simulink model "EV_PV_Charging"  (R2025a)
settings: Solver=ode3  StartTime=0.0  StopTime=1  RelTol=1e-3
PreLoadFcn:
  | %% Parameter file: OBC_4_data.m
  | 
  | %% Model Parameters
  | Ts_Power= 50e-9;        % SPS Model sample time (s)
  | Co=150e-6;              % Output filter (F)
  | Ron_FET=50e-3;          % FET resistance (ohms)
  | Ron_Diode=50e-3;        % FET resistance (ohms)
  | Vf=0.6;                 % Diode forward voltage (V)
  | %
  | %% PFC Data
  | Vnom_ac= 240;           % Nominal Ac voltage (V)
  | Fnom= 60;               % System frequency (Hz)
  | L_PFC= 600e-6;          % PFC Inductance (H)
  | RL_PFC= 20e-3;          % Inductance resistance (Ohm)
  | C_PFC= 2600e-6;         % Capacitance (F)
  | 
  | %% PFC Control System Parameters
  | Ts_Control= 10e-6;      % Control system time (s)
  | Fsw= 100e3;             % PWM Switching frequency (Hz)
  | DT_PFC=400e-9;
  | %
  | % Current Regulator (PR):
  | Kp_I= 0.06;             % Proportional gain
  | Kr_I= 2.5;              % Resonant gain
  | Zeta_I=0.2;             % Damping coefficient
  | Fr_I=Fnom*2;            % Resonant frequency (Hz)
  | %
  | % Voltage Regulator (PI):
  | Kp_V= 0.25;             % Proportional gain
  | Ki_V= 80;               % Integral gain
  | Limit_V= 100;           % Output limit
  | %
  | %% LLC Data
  | Vdc_in=400;             % DC input voltage (V)
  | Vo_nom=400;             % DC nominal output voltage (V)
  | Po_nom=7.2e3;           % Nominal output power (W)
  | Lr=25e-6;               % Transformer leakage inductance (Resonant inductance in Henry)
  | Lm=150e-6;              % Magnetization inductance (H)
  | Cr=75e-9;               % Resonant capacitor (F)
  | Np=10; Ns=12; N=Np/Ns;  % Transformer ratio
  | %
  | %% LLC Control System Parameters
  | DT_LLC=400e-9;
  | Ts_Control=10e-6;
  | % Voltage Regulator (PI):
  | Kp_LLC= 100/4;          % Proportional gain
  | Ki_LLC= 150e3;          % Integral gain
  | fs_LCC_min= 120e3;      % Minimum switching frequency (Hz)
  | fs_LCC_max= 300e3;      % Maximum switching frequency (Hz)
  | Vref_LCC_min= 275;      % Minimum voltage setpoint (V)
  | Vref_LCC_max= 450;      % Maximum voltage setpoint (V)
  | %
  | %%
  | % Resonant tank data
  | Ro=Vo_nom^2/Po_nom      % LLC output load (Ohm)
  | Rac=(8/pi^2)*N^2*Ro     % Equivalent pprimary AC resistance (Ohm)
  | Q=sqrt(Lr/Cr)/Rac       % Quality factor
  | fr=1/(2*pi*sqrt(Lr*Cr)) % Resonant frequency (Hz)
  | m=(Lr+Lm)/Lr            % Ratio of total primary reactance to resonant inductance (Lr)
  | %%
InitFcn:
  | %% Parameter file: OBC_4_data.m
  | 
  | %% Model Parameters
  | Ts_Power= 50e-9;        % SPS Model sample time (s)
  | Co=150e-6;              % Output filter (F)
  | Ron_FET=50e-3;          % FET resistance (ohms)
  | Ron_Diode=50e-3;        % FET resistance (ohms)
  | Vf=0.6;                 % Diode forward voltage (V)
  | %
  | %% PFC Data
  | Vnom_ac= 240;           % Nominal Ac voltage (V)
  | Fnom= 60;               % System frequency (Hz)
  | L_PFC= 600e-6;          % PFC Inductance (H)
  | RL_PFC= 20e-3;          % Inductance resistance (Ohm)
  | C_PFC= 2600e-6;         % Capacitance (F)
  | 
  | %% PFC Control System Parameters
  | Ts_Control= 10e-6;      % Control system time (s)
  | Fsw= 100e3;             % PWM Switching frequency (Hz)
  | DT_PFC=400e-9;
  | %
  | % Current Regulator (PR):
  | Kp_I= 0.06;             % Proportional gain
  | Kr_I= 2.5;              % Resonant gain
  | Zeta_I=0.2;             % Damping coefficient
  | Fr_I=Fnom*2;            % Resonant frequency (Hz)
  | %
  | % Voltage Regulator (PI):
  | Kp_V= 0.25;             % Proportional gain
  | Ki_V= 80;               % Integral gain
  | Limit_V= 100;           % Output limit
  | %
  | %% LLC Data
  | Vdc_in=400;             % DC input voltage (V)
  | Vo_nom=400;             % DC nominal output voltage (V)
  | Po_nom=7.2e3;           % Nominal output power (W)
  | Lr=25e-6;               % Transformer leakage inductance (Resonant inductance in Henry)
  | Lm=150e-6;              % Magnetization inductance (H)
  | Cr=75e-9;               % Resonant capacitor (F)
  | Np=10; Ns=12; N=Np/Ns;  % Transformer ratio
  | %
  | %% LLC Control System Parameters
  | DT_LLC=400e-9;
  | Ts_Control=10e-6;
  | % Voltage Regulator (PI):
  | Kp_LLC= 100/4;          % Proportional gain
  | Ki_LLC= 150e3;          % Integral gain
  | fs_LCC_min= 120e3;      % Minimum switching frequency (Hz)
  | fs_LCC_max= 300e3;      % Maximum switching frequency (Hz)
  | Vref_LCC_min= 275;      % Minimum voltage setpoint (V)
  | Vref_LCC_max= 450;      % Maximum voltage setpoint (V)
  | %
  | %%
  | % Resonant tank data
  | Ro=Vo_nom^2/Po_nom      % LLC output load (Ohm)
  | Rac=(8/pi^2)*N^2*Ro     % Equivalent pprimary AC resistance (Ohm)
  | Q=sqrt(Lr/Cr)/Rac       % Quality factor
  | fr=1/(2*pi*sqrt(Lr*Cr)) % Resonant frequency (Hz)
  | m=(Lr+Lm)/Lr            % Ratio of total primary reactance to resonant inductance (Lr)
  | %%
undefined symbols (not defined in the file or in its folder): D1, Delta, DiscIntNeverNeededParam
libraries: spsSeriesRLCBranchLib x11, spsDiodeLib x7, spsMeanLib x6, MyLibrary x6, spsCurrentMeasurementLib x5, spsVoltageMeasurementLib x5, spsFourierLib x4, spsThreePhaseTransformerTwoWindingsLib x3, spsOnDelayLib x3, spsDistributedParametersLineLib x2, spsThreePhaseParallelRLCLoadLib x2, spsPWMGeneratorDCDCLib x2
(part 4 of 4)

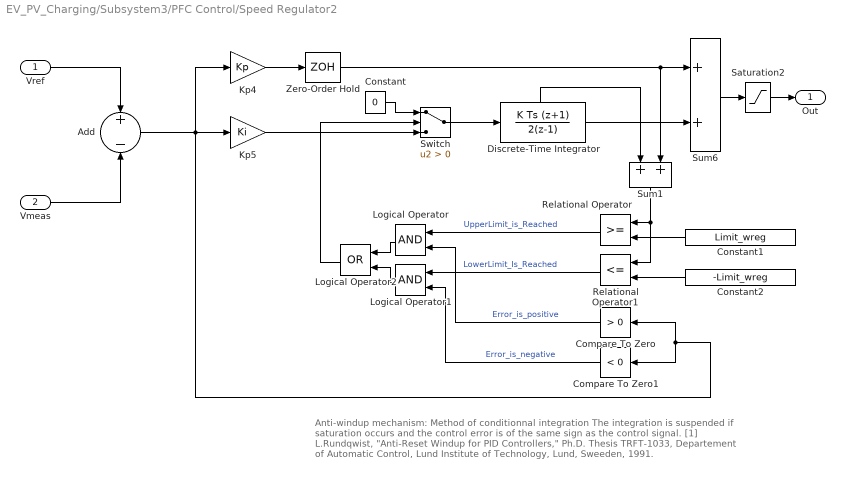
== system EV_PV_Charging/Subsystem3/PFC Control/Speed Regulator2 ==
  note: Anti-windup mechanism: Method of conditionnal integration
      |
      | The integration is suspended if saturation occurs and the
      | control error is of the same sign as the control signal.
      |
      | [1] L.Rundqwist, "Anti-Reset Windup for PID Controllers," Ph.D. Thesis TRFT-1033,
      | Departement of Automatic Control, Lund Institute of Technology, Lund, Sweeden, 1991.
  Vref : Inport  PortDimensions=1
  Vmeas : Inport  Port=2  PortDimensions=1
  Add : Sum  Inputs=+|-
  Compare To Zero : simulink/Logic and Bit Operations/Compare To Zero  relop=>  OutDataTypeStr=uint8  ZeroCross=off
  Compare To Zero1 : simulink/Logic and Bit Operations/Compare To Zero  relop=<  OutDataTypeStr=uint8  ZeroCross=off
  Constant : Constant  Value=0
  Constant1 : Constant  Value=Limit_wreg
  Constant2 : Constant  Value=-Limit_wreg
  Discrete-Time Integrator : DiscreteIntegrator  IntegratorMethod=Integration: Trapezoidal  InitialCondition=Init  SampleTime=Ts  LimitOutput=on  UpperSaturationLimit=Limit_wreg  LowerSaturationLimit=-Limit_wreg  ShowStatePort=on  ICPrevOutput=DiscIntNeverNeededParam  ICPrevScaledInput=DiscIntNeverNeededParam
  Kp4 : Gain  Gain=Kp  SaturateOnIntegerOverflow=on  SampleTime=Ts  OutDataTypeStr=Inherit: Same as input  ParamDataTypeStr=Inherit: Same as input
  Kp5 : Gain  Gain=Ki  SaturateOnIntegerOverflow=on  SampleTime=Ts  OutDataTypeStr=Inherit: Same as input  ParamDataTypeStr=Inherit: Same as input
  Logical Operator : Logic  AllPortsSameDT=off  OutDataTypeStr=boolean
  Logical Operator1 : Logic  AllPortsSameDT=off  OutDataTypeStr=boolean
  Logical Operator2 : Logic  Operator=OR  AllPortsSameDT=off  OutDataTypeStr=boolean
  Relational Operator : RelationalOperator  OutDataTypeStr=boolean  InputSameDT=off
  Relational Operator1 : RelationalOperator  Operator=<=  OutDataTypeStr=boolean  InputSameDT=off
  Saturation2 : Saturate  UpperLimit=Limit_wreg  LowerLimit=-Limit_wreg  SampleTime=Ts
  Sum1 : Sum  InputSameDT=on  SaturateOnIntegerOverflow=on  SampleTime=Ts  OutDataTypeStr=Inherit: Same as first input
  Sum6 : Sum  InputSameDT=on  SaturateOnIntegerOverflow=on  SampleTime=Ts  OutDataTypeStr=Inherit: Same as first input
  Switch : Switch  Criteria=u2 > Threshold  SaturateOnIntegerOverflow=off  InputSameDT=off
  Zero-Order Hold : ZeroOrderHold  SampleTime=Ts
  Out : Outport  SampleTime=Ts  InitialOutput=0  VectorParamsAs1DForOutWhenUnconnected=off
  wires:
  Kp5/1 -> Switch/3
  Switch/1 -> Discrete-Time Integrator/1
  Saturation2/1 -> Out/1
  Discrete-Time Integrator/1 -> Sum6/2
  Kp4/1 -> Zero-Order Hold/1
  Sum6/1 -> Saturation2/1
  Add/1 -> Compare To Zero/1, Compare To Zero1/1, Kp5/1, Kp4/1
  Compare To Zero1/1 -> Logical Operator1/2  "Error_is_negative"
  Logical Operator1/1 -> Logical Operator2/2
  Logical Operator/1 -> Logical Operator2/1
  Compare To Zero/1 -> Logical Operator/2  "Error_is_positive"
  Constant2/1 -> Relational Operator1/2
  Constant1/1 -> Relational Operator/2
  Relational Operator1/1 -> Logical Operator1/1  "LowerLimit_Is_Reached"
  Relational Operator/1 -> Logical Operator/1  "UpperLimit_is_Reached"
  Logical Operator2/1 -> Switch/2
  Sum1/1 -> Relational Operator/1, Relational Operator1/1
  Discrete-Time Integrator/State -> Sum1/1
  Zero-Order Hold/1 -> Sum6/1, Sum1/2
  Constant/1 -> Switch/1
  Vref/1 -> Add/1
  Vmeas/1 -> Add/2
